simulink subsystem "StudentTemplate_SNGKHA008_M2_sim"  (R2025b)
settings: Solver=VariableStepAuto  StartTime=0.0  StopTime=10.0  RelTol=1e-3
libraries: simulink x3, eeGeneralControl x3
(part 2 of 2)

== matlab function StudentTemplate_SNGKHA008_M2_sim/MATLAB Function2 ==
  data: isImuReady input; sensorLeft input; triggerForwardMove output; sensorFront input; sensorRight input; triggerRotation output; rotationAngle output; moveComplete input; turnComplete input; currentRow output; currentCol output; currentHeading output; currentCellWalls output; isLeftWall output; isFrontWall output; isRightWall output; pathStackRows output; pathStackCols output
function [triggerForwardMove, triggerRotation, rotationAngle, ...
          currentRow, currentCol, currentHeading, currentCellWalls, ...
          isLeftWall, isFrontWall, isRightWall, ...
          pathStackRows, pathStackCols] = mazeExplorationController( ...
    isImuReady, sensorLeft, sensorFront, sensorRight, moveComplete, turnComplete)
%#codegen
% Path-based DFS controller:
% - Waits for gyro bias completion (isImuReady) before starting mapping.
% - Stack stores the PATH (breadcrumbs). Top is the previous cell to backtrack to.
% - On forward exploration: push current cell, move to the chosen neighbor.
% - On dead-end: backtrack toward stack top; pop AFTER the backtrack move completes.
% - Robust wall mirroring; clean turn→move handoff with 1-tick cooldown after turns.
% - NEW: After each one-block forward move completes, wait POST_MOVE_PAUSE_DURATION.
%% ---- Tunables ----
WALL_DETECT_DISTANCE   = 0.15;     % [m]
ANGLE_CLOCKWISE        = -pi/2;    % CW (right)
ANGLE_COUNTER_CLOCKWISE =  pi/2;    % CCW (left)
ANGLE_REVERSE          =  pi;      % 180
MAZE_ROWS              = uint8(4);
MAZE_COLS              = uint8(6);
START_ROW              = uint8(MAZE_ROWS); % bottom-left row
START_COL              = uint8(1);          % leftmost col
SENSOR_SETTLE_DURATION = uint8(2);
% NEW: post-move wait
POST_MOVE_PAUSE_DURATION = uint16(10);
%% ---- Cast inputs ----
isImuReady = (isImuReady ~= 0);
sensorLeft   = double(sensorLeft);
sensorFront  = double(sensorFront);
sensorRight  = double(sensorRight);
moveComplete   = (moveComplete ~= 0);
turnComplete   = (turnComplete ~= 0);
%% ---- Default outputs ----
triggerForwardMove = 0.0; triggerRotation = 0.0; rotationAngle = 0.0;
currentRow = 0.0; currentCol = 0.0; currentHeading = 0.0; currentCellWalls = uint8(0);
isLeftWall  = double(sensorLeft  < WALL_DETECT_DISTANCE);
isFrontWall = double(sensorFront < WALL_DETECT_DISTANCE);
isRightWall = double(sensorRight < WALL_DETECT_DISTANCE);
% Last-5 stack preview (top-most first). 0 = no entry.
pathStackRows = zeros(1,5);  % doubles for scope
pathStackCols = zeros(1,5);
%% ---- Persistent state ----
persistent isInitialized ...
           visitedCells wallMap ...
           robotRow robotCol robotHeading ...
           pathStackRow pathStackCol pathStackPointer ...
           needsSensing sensorSettleTimer ...
           robotState pendingRotationAngle sendMovePulse sendTurnPulse ...
           hasJustTurned ...
           hasNextTarget targetRow targetCol isBacktracking ...
           hasStarted ...
           postMovePauseTimer   % <<< NEW
if isempty(isInitialized)
    visitedCells = false(double(MAZE_ROWS), double(MAZE_COLS));
    % wallMap(:,:,d+1): 1=N, 2=E, 3=S, 4=W
    wallMap      = false(double(MAZE_ROWS), double(MAZE_COLS), 4);
    robotRow     = START_ROW;
    robotCol     = START_COL;
    robotHeading = uint8(1);   % 0=N,1=E,2=S,3=W (start East)
    MAX_STACK_DEPTH = uint32(double(MAZE_ROWS) * double(MAZE_COLS));
    pathStackRow = zeros(double(MAX_STACK_DEPTH),1,'uint8');
    pathStackCol = zeros(double(MAX_STACK_DEPTH),1,'uint8');
    pathStackPointer = uint16(0);
    needsSensing    = true;
    sensorSettleTimer = uint8(0);
    robotState      = uint8(0); % 0=IDLE,1=MOVING,2=TURNING
    pendingRotationAngle = 0.0;
    sendMovePulse   = false;
    sendTurnPulse   = false;
    hasJustTurned   = false;
    hasNextTarget   = false;
    targetRow       = uint8(0);
    targetCol       = uint8(0);
    isBacktracking  = false;
    hasStarted = false;   % wait for isImuReady
    postMovePauseTimer = uint16(0); % <<< NEW
    isInitialized = true;
end
%% ---- STARTUP GATE: wait for gyro bias ready ----
if ~hasStarted
    if isImuReady
        hasStarted    = true;
        needsSensing  = true;
        sensorSettleTimer = uint8(0);
    else
        % Hold outputs steady, do NOT sense/map/move yet
        triggerForwardMove = 0.0; triggerRotation = 0.0; rotationAngle = pendingRotationAngle;
        currentRow = double(robotRow);
        currentCol = double(robotCol);
        currentHeading = double(robotHeading);
        currentCellWalls = uint8(0);      % unknown before mapping
        % stack preview
        stackPtr = double(pathStackPointer);
        for i=1:5
            idx = stackPtr-(i-1);
            if idx>=1
                pathStackRows(i) = double(pathStackRow(idx));
                pathStackCols(i) = double(pathStackCol(idx));
            else
                pathStackRows(i) = 0; pathStackCols(i) = 0;
            end
        end
        return;
    end
end
%% ---- GLOBAL POST-MOVE WAIT GATE (highest priority after startup) ----
if postMovePauseTimer > 0
    postMovePauseTimer = postMovePauseTimer - 1;
    % Freeze planning/sensing/commands during wait
    triggerForwardMove = 0.0; triggerRotation = 0.0; rotationAngle = pendingRotationAngle;
    currentRow   = double(robotRow);
    currentCol   = double(robotCol);
    currentHeading = double(robotHeading);
    currentCellWalls = uint8(wallMap(robotRow,robotCol,1)) ...
                   + bitshift(uint8(wallMap(robotRow,robotCol,2)),1) ...
                   + bitshift(uint8(wallMap(robotRow,robotCol,3)),2) ...
                   + bitshift(uint8(wallMap(robotRow,robotCol,4)),3);
    % Stack preview
    stackPtr = double(pathStackPointer);
    for i=1:5
        idx = stackPtr-(i-1);
        if idx>=1
            pathStackRows(i) = double(pathStackRow(idx));
            pathStackCols(i) = double(pathStackCol(idx));
        else
            pathStackRows(i) = 0; pathStackCols(i) = 0;
        end
    end
    return;
end
%% ---- Helpers ----
    function tf = isWithinGrid(r, c)
        tf = (r>=1) && (r<=double(MAZE_ROWS)) && ...
             (c>=1) && (c<=double(MAZE_COLS));
    end
    function [dr,dc] = getDirectionVector(dir)
        switch dir
            case 0, dr = -1; dc =  0; % N
            case 1, dr =  0; dc =  1; % E
            case 2, dr =  1; dc =  0; % S
            otherwise, dr = 0; dc = -1; % W
        end
    end
    function opp = getOppositeDirection(dir), opp = uint8(mod(double(dir)+2,4)); end
    function empty = isPathStackEmpty(), empty = (pathStackPointer==0); end
    function pushToPathStack(r, c)
        pathStackPointer = pathStackPointer + 1;
        pathStackRow(pathStackPointer) = uint8(r);
        pathStackCol(pathStackPointer) = uint8(c);
    end
    function [r, c] = peekPathStack()
        r = pathStackRow(pathStackPointer); c = pathStackCol(pathStackPointer);
    end
    function popFromPathStack()
        if pathStackPointer>0, pathStackPointer = pathStackPointer - 1; end
    end
    function dabs = getAbsoluteDirectionTo(r, c)
        if (double(r)==double(robotRow)-1) && (double(c)==double(robotCol))
            dabs = uint8(0);   % N
        elseif (double(r)==double(robotRow)) && (double(c)==double(robotCol)+1)
            dabs = uint8(1);   % E
        elseif (double(r)==double(robotRow)+1) && (double(c)==double(robotCol))
            dabs = uint8(2);   % S
        else
            dabs = uint8(3);   % W
        end
    end
    function ang = getRelativeAngle(currentDir, desiredDir)
        leftDir  = uint8(mod(double(currentDir)+3,4)); % CCW
        rightDir = uint8(mod(double(currentDir)+1,4)); % CW
        backDir  = uint8(mod(double(currentDir)+2,4));
        if     desiredDir == currentDir, ang = 0.0;
        elseif desiredDir == leftDir,  ang =  ANGLE_COUNTER_CLOCKWISE;
        elseif desiredDir == rightDir, ang =  ANGLE_CLOCKWISE;
        elseif desiredDir == backDir,  ang =  ANGLE_REVERSE;
        else
            d = double(mod(double(desiredDir) - double(currentDir),4));
            if d == 1, ang = ANGLE_CLOCKWISE;
            elseif d==2, ang = ANGLE_REVERSE;
            else,        ang = ANGLE_COUNTER_CLOCKWISE;
            end
        end
    end
    function recordWall(r, c, absDir)
        wallMap(r, c, absDir+1) = true;
        [dr,dc] = getDirectionVector(absDir);
        rn = double(r)+dr; cn = double(c)+dc;
        if isWithinGrid(rn,cn)
            wallMap(rn, cn, getOppositeDirection(absDir)+1) = true;
        end
    end
%% ---- Sense when idle & settled ----
dir_front = uint8(0); dir_left = uint8(0); dir_right = uint8(0); dir_back = uint8(0);
nl = 0.0; ml = 0.0; nf = 0.0; mf = 0.0; nr = 0.0; mr = 0.0; nb = 0.0; mb = 0.0;
if needsSensing && (robotState == uint8(0))
    if sensorSettleTimer > 0
        sensorSettleTimer = sensorSettleTimer - 1;
        rotationAngle = pendingRotationAngle;
        currentRow   = double(robotRow);
        currentCol   = double(robotCol);
        currentHeading = double(robotHeading);
        currentCellWalls = uint8(wallMap(robotRow,robotCol,1)) ...
                       + bitshift(uint8(wallMap(robotRow,robotCol,2)),1) ...
                       + bitshift(uint8(wallMap(robotRow,robotCol,3)),2) ...
                       + bitshift(uint8(wallMap(robotRow,robotCol,4)),3);
        % Stack preview
        stackPtr = double(pathStackPointer);
        for i=1:5
            idx = stackPtr-(i-1);
            if idx>=1
                pathStackRows(i) = double(pathStackRow(idx));
                pathStackCols(i) = double(pathStackCol(idx));
            else
                pathStackRows(i) = 0; pathStackCols(i) = 0;
            end
        end
        return;
    end
    visitedCells(robotRow,robotCol) = true;
    dir_front = robotHeading;
    dir_left  = uint8(mod(double(robotHeading)+3,4));
    dir_right = uint8(mod(double(robotHeading)+1,4));
    if sensorFront < WALL_DETECT_DISTANCE, recordWall(robotRow,robotCol,dir_front); end
    if sensorLeft  < WALL_DETECT_DISTANCE, recordWall(robotRow,robotCol,dir_left ); end
    if sensorRight < WALL_DETECT_DISTANCE, recordWall(robotRow,robotCol,dir_right); end
    hasNextTarget  = false;
    isBacktracking = false;
    needsSensing   = false;
    sensorSettleTimer = SENSOR_SETTLE_DURATION;
end
%% ---- Planner / Controller FSM ----
if isempty(hasJustTurned), hasJustTurned = false; end
switch robotState
    case uint8(0) % IDLE
        if hasJustTurned
            hasJustTurned = false;
            % stack preview
            stackPtr = double(pathStackPointer);
            for i=1:5
                idx = stackPtr-(i-1);
                if idx>=1
                    pathStackRows(i) = double(pathStackRow(idx));
                    pathStackCols(i) = double(pathStackCol(idx));
                else
                    pathStackRows(i) = 0; pathStackCols(i) = 0;
                end
            end
            return;
        end
        dir_front = robotHeading;
        dir_left  = uint8(mod(double(robotHeading)+3,4));
        dir_right = uint8(mod(double(robotHeading)+1,4));
        dir_back  = uint8(mod(double(robotHeading)+2,4));
        if hasNextTarget
            dabs = getAbsoluteDirectionTo(targetRow, targetCol);
            ang  = getRelativeAngle(robotHeading, dabs);
            if abs(ang) < 1e-9
                if ~isBacktracking, pushToPathStack(robotRow, robotCol); end
                pendingRotationAngle = 0.0; sendMovePulse = true; robotState = uint8(1);
            else
                pendingRotationAngle = ang;  sendTurnPulse = true; robotState = uint8(2);
            end
            return;
        end
        [drl,dcl] = getDirectionVector(dir_left);   nl = double(robotRow)+drl; ml = double(robotCol)+dcl;
        [drf,dcf] = getDirectionVector(dir_front);  nf = double(robotRow)+drf; mf = double(robotCol)+dcf;
        [drr,dcr] = getDirectionVector(dir_right);  nr = double(robotRow)+drr; mr = double(robotCol)+dcr;
        L_open = ~wallMap(robotRow,robotCol,dir_left +1)  && isWithinGrid(nl,ml);
        F_open = ~wallMap(robotRow,robotCol,dir_front+1)  && isWithinGrid(nf,mf);
        R_open = ~wallMap(robotRow,robotCol,dir_right+1)  && isWithinGrid(nr,mr);
        choseForward = false;
        if F_open && ~visitedCells(nf,mf)
            targetRow = uint8(nf); targetCol = uint8(mf);
            hasNextTarget = true; isBacktracking = false; choseForward = true;
        elseif L_open && ~visitedCells(nl,ml)
            targetRow = uint8(nl); targetCol = uint8(ml);
            hasNextTarget = true; isBacktracking = false; choseForward = true;
        elseif R_open && ~visitedCells(nr,mr)
            targetRow = uint8(nr); targetCol = uint8(mr);
            hasNextTarget = true; isBacktracking = false; choseForward = true;
        end
        if ~choseForward
            if ~isPathStackEmpty()
                [pr,pc] = peekPathStack();
                targetRow = pr; targetCol = pc;
                hasNextTarget = true; isBacktracking = true;
            else
                hasNextTarget = false;
            end
        end
        if hasNextTarget
            dabs = getAbsoluteDirectionTo(targetRow, targetCol);
            ang  = getRelativeAngle(robotHeading, dabs);
            if abs(ang) < 1e-9
                if ~isBacktracking, pushToPathStack(robotRow, robotCol); end
                pendingRotationAngle = 0.0; sendMovePulse = true; robotState = uint8(1);
            else
                pendingRotationAngle = ang;  sendTurnPulse = true; robotState = uint8(2);
            end
        end
    case uint8(1) % MOVING
        if moveComplete
            % Update position in the direction of current heading.
            [drm,dcm] = getDirectionVector(robotHeading);
            robotRow = uint8(max(1, min(double(MAZE_ROWS), double(robotRow)+drm)));
            robotCol = uint8(max(1, min(double(MAZE_COLS), double(robotCol)+dcm)));
            if isBacktracking && ~isPathStackEmpty()
                popFromPathStack();
            end
            hasNextTarget  = false;
            isBacktracking = false;
            % NEW: start post-move wait window
            postMovePauseTimer = POST_MOVE_PAUSE_DURATION;
            % Prepare next sense AFTER wait ends
            needsSensing  = true;
            sensorSettleTimer = SENSOR_SETTLE_DURATION;
            robotState    = uint8(0);
        end
    case uint8(2) % TURNING
        if turnComplete
            if abs(pendingRotationAngle) < 1e-9
                % no change
            elseif abs(pendingRotationAngle - ANGLE_COUNTER_CLOCKWISE)  < 1e-6
                robotHeading = uint8(mod(double(robotHeading)+3,4)); % CCW
            elseif abs(pendingRotationAngle - ANGLE_CLOCKWISE)   < 1e-6
                robotHeading = uint8(mod(double(robotHeading)+1,4)); % CW
            else
                robotHeading = uint8(mod(double(robotHeading)+2,4)); % 180
            end
            robotState = uint8(0);
            hasJustTurned = true;   % one tick cooldown
        end
end
%% ---- Emit pulses ----
if sendMovePulse, triggerForwardMove = 1.0; sendMovePulse = false; end
if sendTurnPulse, triggerRotation = 1.0; sendTurnPulse = false; end
%% ---- Debug / held outputs ----
rotationAngle = pendingRotationAngle;
currentRow   = double(robotRow);
currentCol   = double(robotCol);
currentHeading = double(robotHeading);
currentCellWalls = uint8(wallMap(robotRow,robotCol,1)) ...
               + bitshift(uint8(wallMap(robotRow,robotCol,2)),1) ...
               + bitshift(uint8(wallMap(robotRow,robotCol,3)),2) ...
               + bitshift(uint8(wallMap(robotRow,robotCol,4)),3);
% Stack preview (top-most first)
stackPtr = double(pathStackPointer);
for i=1:5
    idx = stackPtr-(i-1);
    if idx>=1
        pathStackRows(i) = double(pathStackRow(idx));
        pathStackCols(i) = double(pathStackCol(idx));
    else
        pathStackRows(i) = 0; pathStackCols(i) = 0;
    end
end
end

== matlab function StudentTemplate_SNGKHA008_M2_sim/MATLAB Function3 ==
  settings: updateMethod=DISCRETE
  data: gyroRate input; enable input; estimatedBias output; isBiasReady output
function [estimatedBias, isBiasReady] = calculateGyroBias(gyroRate, enable)
%#codegen
persistent sampleCounter;
persistent sumAccumulator;        % Persistent accumulator

if isempty(sampleCounter)
    sampleCounter = 0;
    sumAccumulator = 0.0;
end

if enable < 0.5
    isBiasReady = 0;
    estimatedBias = 0.0;
    % Reset persistent state
    sumAccumulator = 0.0;
    sampleCounter = 0;
    return;
end

if sampleCounter < 1000
    sampleCounter = sampleCounter + 1;
    sumAccumulator = sumAccumulator + gyroRate;
    isBiasReady = 0;
    estimatedBias = 0.0; % Bias is not ready yet
else
    isBiasReady = 1;
    % Calculate the average bias
    estimatedBias = sumAccumulator / double(sampleCounter);
end

== matlab function StudentTemplate_SNGKHA008_M2_sim/mapMaze ==
  settings: updateMethod=DISCRETE
  data: robotX_m output; leftEncoderPulse input; robotY_m output; rightEncoderPulse input; isSpinning input; imuHeadingRad input; robotHeading_rad output; gridCol output; gridRow output; visitCountMap output; isTaskComplete output
function [robotX_m, robotY_m, robotHeading_rad, gridCol, gridRow, visitCountMap, isTaskComplete] = updatePoseAndGrid( ...
    leftEncoderPulse, rightEncoderPulse, isSpinning, imuHeadingRad)
% takes in left and right encoder pulses and returns the mouse's relative
% position and index in the maze
% constants
WHEEL_RADIUS_M  = 0.031;        % wheel radius (m)
HALF_AXLE_WIDTH_M = 0.060;  % half axle length (m)
WHEELBASE_M = 2*HALF_AXLE_WIDTH_M;
TICKS_PER_REV = 8;              % ticks per revolution
CELL_SIZE_M = 0.20;     % maze cell size (m)
GRID_COLS = 6; GRID_ROWS = 4; % grid dims (x cols, y rows)
% persistent state
persistent currentX currentY currentTheta lastLeftPulse lastRightPulse cellVisitCounts lastGridCol lastGridRow
if isempty(currentX)
    currentX = 0.1; currentY = 0.1; currentTheta = 0;   % initial position
    lastLeftPulse = false; lastRightPulse = false; % previous pulse sample for edge detect
    cellVisitCounts = zeros(GRID_ROWS, GRID_COLS);  % initialize map
    lastGridCol = 0;
    lastGridRow = 0;
end
% rising-edge detection
leftEdgeDetected = (leftEncoderPulse > 0.5) && (lastLeftPulse <= 0.5);
rightEdgeDetected = (rightEncoderPulse > 0.5) && (lastRightPulse <= 0.5);
% update prev ticks
lastLeftPulse = leftEncoderPulse;
lastRightPulse = rightEncoderPulse;
%  edge count (0 or 1)
leftTickCount = double(leftEdgeDetected);
rightTickCount = double(rightEdgeDetected);
% SIGNS: when reversing (spinning)
if isSpinning == 1
    leftSign = +1;
    rightSign = -1;
else
    leftSign = +1;
    rightSign = +1;
end
% angular displacement of wheels (rad)
leftWheelRad = leftSign * (2*pi/TICKS_PER_REV) * (leftTickCount);
rightWheelRad = rightSign * (2*pi/TICKS_PER_REV) * (rightTickCount);
% Linear and angular velocity (eqn 15 and 16)
distanceDelta_m = WHEEL_RADIUS_M/2 * (rightWheelRad + leftWheelRad); % forward displacement
%dth = WHEEL_RADIUS_M / WHEELBASE_M * (rightWheelRad - leftWheelRad); % angular displacement - TICKS
currentTheta = imuHeadingRad; % GYRO
% Pose update using robot kinematics in inertial frame (eq 20)
deltaX = distanceDelta_m * cos(currentTheta);
deltaY = distanceDelta_m * sin(currentTheta);
currentX = currentX + deltaX;
currentY = currentY + deltaY;
%currentTheta = currentTheta + dth; %TICKS
% convert position to relative idex for map matrix
gridCol = min(max(floor(currentX / CELL_SIZE_M) + 1, 1), GRID_COLS);
gridRow = min(max(floor(currentY / CELL_SIZE_M) + 1, 1), GRID_ROWS);
% increment visit counter (only if in new cell)
if (gridCol ~= lastGridCol) || (gridRow ~= lastGridRow)
    cellVisitCounts(gridRow, gridCol) = cellVisitCounts(gridRow, gridCol) + 1;
    lastGridCol = gridCol;
    lastGridRow = gridRow;
end
% check if mapping is done
if cellVisitCounts(1:1) > 1
    isTaskComplete = 1;
else
    isTaskComplete = 0;
end
% outputs visit matrix flipped
visitCountMap = flipud(cellVisitCounts);
% outputs
robotX_m = currentX;
robotY_m = currentY;
robotHeading_rad = currentTheta;
end

== stateflow chart StudentTemplate_SNGKHA008_M2_sim/Chart ==
  state Reverse
    entry:
    isReversed = false;
    during:
    if (Reverse >=3.14)
    isReversed = true;
    elseif (Reverse <= -3.14)
    isReversed = true;
    else
    isReversed = false;
    end
  (default) -> Reverse
  data: Reverse input; isReversed output

== matlab function StudentTemplate_SNGKHA008_M2_sim/YawCorrection/AntiWindup ==
  settings: updateMethod=DISCRETE
  data: AngleError input; intError output
function intError  = Anti_Windup( AngleError)
persistent prevIntError
if isempty(prevIntError)
    prevIntError = 0;
end
prevIntError = prevIntError + AngleError;
intError = max(min(prevIntError,100),-100);

== matlab function StudentTemplate_SNGKHA008_M2_sim/MATLAB Function4 ==
  settings: updateMethod=DISCRETE
  data: tof_Right input; correction output
function correction = TOF_Correction(tof_Right)
% TOF_RightCorrection - Maintain straight motion using right TOF sensor feedback

    targetDist = 0.078;   % Desired right wall distance (m)
    Kp = 70;              % Proportional gain
    Ki = 1;             % Integral gain
    alpha = 0.05;         % Integration smoothing factor (acts like dt)
    intLimit = 100;       % Anti-windup limit for the integrator

    persistent intError
    if isempty(intError)
        intError = 0;
    end

    
    error = targetDist - tof_Right;   % Positive means too close to wall on right

    
    intError = intError + alpha * error;
    intError = max(min(intError, intLimit), -intLimit);

    correction = Kp * error + Ki * intError;
end

== stateflow chart StudentTemplate_SNGKHA008_M2_sim/speedCorrection ==
  state tofSmallerThan1
    v_Left=baseSpeed-correction-abs(TOF_correction);
    v_Right= baseSpeed;
  state AngleGreaterThan0
    v_Left = baseSpeed - correction
    v_Right = baseSpeed
  state AngleIsZero
    v_Left = baseSpeed
    v_Right =baseSpeed
  state AngleLessThan0
    v_Left = baseSpeed
    v_Right = baseSpeed - correction
  state tofBiggerThan1
    v_Left=baseSpeed-correction + abs(TOF_correction);
    v_Right= baseSpeed-abs(TOF_correction);
  state tofSmaller
    v_Left=baseSpeed- abs(TOF_correction)
    v_Right= baseSpeed-correction
  state tofBigger
    v_Left=baseSpeed
    v_Right= baseSpeed-correction- abs(TOF_correction)
  (default) -> AngleIsZero
  AngleGreaterThan0 -> tofSmallerThan1 [order 2] : [Turn ==0 && TOF_R <0.078]
  AngleIsZero -> AngleGreaterThan0 [order 1] : [Angle>0]
  tofSmallerThan1 -> AngleGreaterThan0 : [ TOF_R >=0.078]
  AngleIsZero -> AngleLessThan0 [order 2] : [Angle<0]
  AngleGreaterThan0 -> tofBiggerThan1 [order 1] : [Turn==0 && TOF_R >0.078]
  tofBiggerThan1 -> AngleGreaterThan0 : [ TOF_R <= 0.078]
  AngleLessThan0 -> tofSmaller [order 2] : [TOF_R <0.078]
  AngleLessThan0 -> tofBigger [order 1] : [TOF_R >0.078]
  tofBigger -> AngleLessThan0 : [TOF_R <= 0.078]
  tofSmaller -> AngleLessThan0 : [TOF_R >=0.078]
  data: correction input; Angle input; v_Left output; v_Right output; TOF_correction input; TOF_R input; Turn input; baseSpeed input

== stateflow chart StudentTemplate_SNGKHA008_M2_sim/Chart1 ==
  settings: updateMethod=DISCRETE  sampleTime=0.005
  state Move
    lPrevious = v_Left;
    rPrevious = v_Right;
    Omega_R = rPrevious;
    Omega_L = lPrevious;
    turn_dir=0;
    priority = 1;
    deadend= 1;
  state wait
  state TurnLeft1
    Omega_R=rPrevious;
    Omega_L=0;
    turn_dir = 1;
  state AfterLeftTurn1
    Omega_R =0;
    Omega_L =0;
    turn_dir=0;
  state TurnLeft
    Omega_R=rPrevious;
    Omega_L=0;
    turn_dir = 1;
  state AfterTurn
    Omega_R = 0;
    Omega_L = 0;
    turn_dir = 0;
  state wait1
  state AfterRightTurn
    Omega_R =0;
    Omega_L =0;
    turn_dir =0;
  state TurnRight
    Omega_R=0;
    Omega_L=lPrevious;
    turn_dir = 1;
  state Continue
    Omega_R = rPrevious;
    Omega_L = lPrevious;
    turn_dir = 0;
  state DeadEnd
    Omega_R = -rPrevious;
    Omega_L = lPrevious;
    deadend = 0;
    turn_dir = 1;
  state DeadEnd1
    Omega_R = -rPrevious;
    Omega_L = lPrevious;
    deadend = 1;
    turn_dir = 1;
  state Complete
    turn_dir =0;
    Omega_R =0;
    Omega_L = 0;
  AfterLeftTurn1 -> TurnLeft [order 2] : [tof_Front<=0.11 && tof_Left >=0.25]
  (default) -> Move
  wait -> TurnLeft : [after(0.5,sec)]
  Move -> wait [order 2] : [tof_Left>=0.25 && tof_Front >0.11]
  TurnLeft -> AfterTurn : [abs(Angle)>=1.567]
  TurnLeft1 -> AfterLeftTurn1 : [abs(Angle)>= 1.567]
  Move -> TurnLeft [order 1] : [tof_Front<=0.10 && tof_Left>=0.25]
  wait1 -> TurnLeft1 : [after(0.5,sec)]
  AfterRightTurn -> TurnLeft [order 2] : [tof_Front<=0.1 && tof_Left >=0.25]
  AfterLeftTurn1 -> TurnRight [order 3] : [tof_Front<=0.11 && tof_Right>=0.25]
  AfterLeftTurn1 -> Continue [order 1] : [after(0.1,sec)]
  AfterTurn -> Continue : [after(0.1,sec)]
  Continue -> wait1 [order 2] : [tof_Left>=0.25 && tof_Front >0.11]
  TurnRight -> AfterRightTurn : [abs(Angle)>=1.567]
  Continue -> TurnRight [order 3] : [tof_Front <=0.11 && tof_Right>=0.25]
  AfterRightTurn -> Continue [order 1] : [after(0.1,sec)]
  Continue -> DeadEnd [order 1] : [tof_Front <=0.09 && tof_Left <0.25 && tof_Right < 0.25 && deadend ==1]
  DeadEnd1 -> Continue : [abs(Angle)>=1.567]
  DeadEnd -> Complete : [abs(Angle) >= 1.567]
  Complete -> DeadEnd1
  data: Omega_R output; Omega_L output; tof_Front input; v_Left input; Angle input; v_Right input; lPrevious local; rPrevious local; turn_dir output; tof_Left input; tof_Right input; priority local; deadend local

== stateflow chart StudentTemplate_SNGKHA008_M2_sim/Chart2 ==
  state PreTurn
    entry:
    state_out = 2;
    v = 0.6*(30);
    yaw_ref = corridor_heading + turn_dir* pi/2;
    during:
    v_r = v;
    v_l = v;
  state WallFollow_
    entry:
    state_out = 1;
    v = 30;
    during:
    e = tof_right - 0.4;
    de = (e - e_prev) / dt;
    omega = Kp * e + Kd * de;
    v_r = v + (b/2) * omega;
    v_l = v - (b/2) * omega;
    e_prev = e;
    corridor_heading = yaw;
  state ExecuteTurn
    entry:
    state_out = 3;
    during:
    yaw_err = yaw_ref - yaw;
    omega = Kp_turn*yaw_err;
    v_r =  (30) * 0.5 + (b/2)*omega;
    v_l =  (30) * 0.5 - (b/2)*omega;
  state Align
    entry:
    state_out = 4;
    during:
    e = tof_right - 0.4;
    if abs(e) > 0.01
    omega = K_align * e;
    else
    omega = 0;
    end
    v_r = (30)*0.4 + (b/2)*omega;
    v_l = (30)*0.4 - (b/2)*omega;
    exit:
    corridor_heading = yaw;
  (default) -> WallFollow_
  PreTurn -> ExecuteTurn : [tof_front < 0.15 || tof_left>0.1 || tof_right>0.1]
  WallFollow_ -> PreTurn : [tof_front < 0.15 || tof_left>0.1 || tof_right> 0.1]
  Align -> WallFollow_ : [after(0.3, sec) || abs(e) < 0.01 && abs(yaw_err) < deg2rad(3)]
  ExecuteTurn -> Align : after(0.1, sec)[(abs(yaw_err) < deg2rad(3)) ]
  data: K_align input; Kd input; Kp input; Kp_turn input; b input; dt input; tof_front input; tof_right input; turn_dir input; yaw input; v_l output; v_r output; de local; e local =0; e_prev local =0; omega local; v local; yaw_err local =0; yaw_ref local; state_out output; tof_left input; d_open local; wall_thresh local; corridor_heading output =0

== matlab function StudentTemplate_SNGKHA008_M2_sim/MATLAB Function5 ==
  data: tof_front input; tof_left input; turn_dir output; tof_right input; d_open input; wall_thresh input

function turn_dir = detectTurn(tof_front, tof_left, tof_right, d_open, wall_thresh)
% Returns turn_dir:
%   +1 = turn left
%   -1 = turn right
%    0 = go straight

turn_dir = 0; % default

% === CASE 1: Wall in front ===
if tof_front < d_open
    if tof_right < wall_thresh && tof_left > wall_thresh
        turn_dir = 1; % Left clear, right blocked → turn left
    elseif tof_left < wall_thresh && tof_right > wall_thresh
        turn_dir = -1; % Right clear, left blocked → turn right
    elseif tof_right > wall_thresh && tof_left > wall_thresh
        % Both sides open (junction) — pick one
        turn_dir = 1; % e.g. prefer left (can randomize later)
    else
        % Dead end → turn around
        turn_dir = 1; % or pick a default 180° turn
    end

% === CASE 2: Front clear, but a side opens ===
elseif tof_right > d_open && tof_left < wall_thresh
    turn_dir = -1; % opening on right while hugging left wall
elseif tof_left > d_open && tof_right < wall_thresh
    turn_dir = 1; % opening on left while hugging right wall

% === CASE 3: Everything normal ===
else
    turn_dir = 0; % continue straight
end

end
